simulink model "testSHM"  (Simulink 7.2)
settings: Solver=ode1  StartTime=0.0  StopTime=10.0  FixedStep=0.001  RelTol=1e-3
libraries: rtai_devices x1
settings Model: Creator=johannes  LastModifiedBy=johannes
settings RTWCC: SystemTargetFile=rtai.tlc  GenCodeOnly=on  TemplateMakefile=rtai.tmf  Description=Linux RTAI Real-Time Target  ProcessScript=rtai_make_rtw_hook
settings STFCustomTargetCC: ModelReferenceCompliant=off  MatFileLogging=on  SystemTargetFile=rtai.tlc

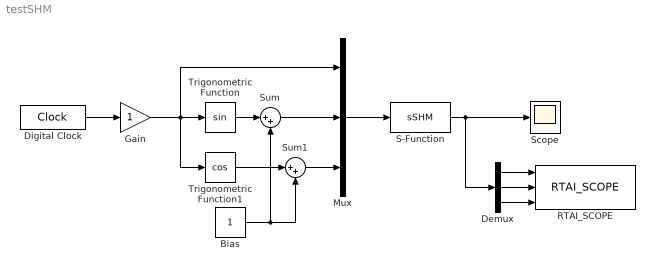
== system testSHM ==
  Bias : Constant  OutDataType=sfix(16)  OutScaling=2^0
  Demux : Demux  Outputs=3
  Digital Clock : DigitalClock  SampleTime=0.001
  Gain : Gain  ParameterDataType=sfix(16)  ParameterScaling=2^0  OutDataType=sfix(16)  OutScaling=2^0
  Mux : Mux  Inputs=3
  RTAI_SCOPE : rtai_devices/RTAI_SCOPE  numch=3  ts=-1
  S-Function : S-Function  FunctionName=sSHM  EnableBusSupport=off
  Scope : Scope
  Sum : Sum  Inputs=|++  OutDataType=sfix(16)  OutScaling=2^0
  Sum1 : Sum  Inputs=|++  OutDataType=sfix(16)  OutScaling=2^0
  Trigonometric Function : Trigonometry
  Trigonometric Function1 : Trigonometry  Operator=cos
  wires:
  Digital Clock/1 -> Gain/1
  Mux/1 -> S-Function/1
  Gain/1 -> Trigonometric Function/1, Trigonometric Function1/1, Mux/1
  Trigonometric Function/1 -> Sum/1
  Trigonometric Function1/1 -> Sum1/1
  Sum1/1 -> Mux/3
  Sum/1 -> Mux/2
  Bias/1 -> Sum1/2, Sum/2
  S-Function/1 -> Scope/1, Demux/1
  Demux/1 -> RTAI_SCOPE/1
  Demux/2 -> RTAI_SCOPE/2
  Demux/3 -> RTAI_SCOPE/3
